simulink subsystem "CheckInput_Bypass"  (R2021a)
settings: Solver=VariableStepAuto  StartTime=0.0  StopTime=10.0  RelTol=1e-3
undefined symbols (not defined in the file): ErrVarCheckIn
settings Model: Creator=zurnmar  LastModifiedBy=zurnmar

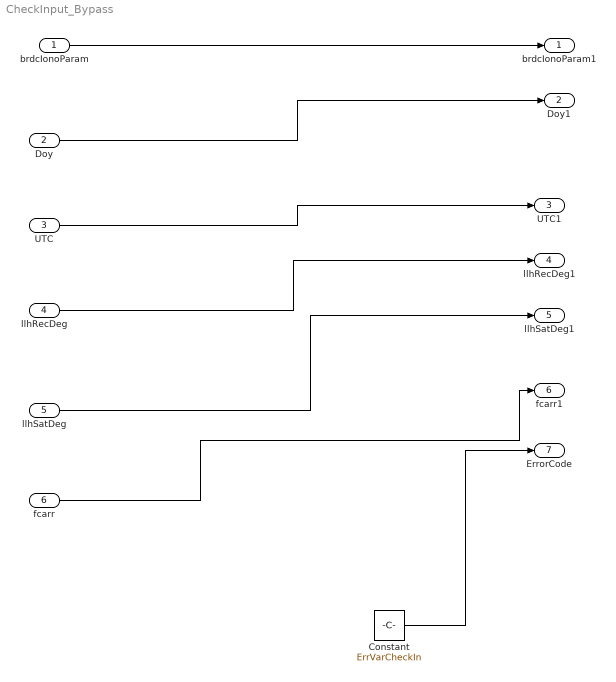
== system CheckInput_Bypass ==
  brdcIonoParam : Inport  PortDimensions=[3,1]
  Doy : Inport  Port=2  PortDimensions=1
  UTC : Inport  Port=3  PortDimensions=1
  llhRecDeg : Inport  Description=dxdxxdxhx  Port=4  PortDimensions=[3,1]
  llhSatDeg : Inport  Port=5  PortDimensions=[3,1]
  fcarr : Inport  Port=6  PortDimensions=1
  Constant : Constant  Value=ErrVarCheckIn  VectorParams1D=off  OutDataTypeStr=uint16
  brdcIonoParam1 : Outport
  Doy1 : Outport  Port=2
  UTC1 : Outport  Port=3
  llhRecDeg1 : Outport  Port=4
  llhSatDeg1 : Outport  Port=5
  fcarr1 : Outport  Port=6
  ErrorCode : Outport  Port=7
  wires:
  brdcIonoParam/1 -> brdcIonoParam1/1
  Doy/1 -> Doy1/1
  UTC/1 -> UTC1/1
  llhRecDeg/1 -> llhRecDeg1/1
  llhSatDeg/1 -> llhSatDeg1/1
  fcarr/1 -> fcarr1/1
  Constant/1 -> ErrorCode/1
